simulink model "sym_uklad_D"  (R2024b)
settings: Solver=VariableStepAuto  StartTime=0.0  StopTime=0.01  RelTol=1e-3
settings Model: Creator=User  LastModifiedBy=User

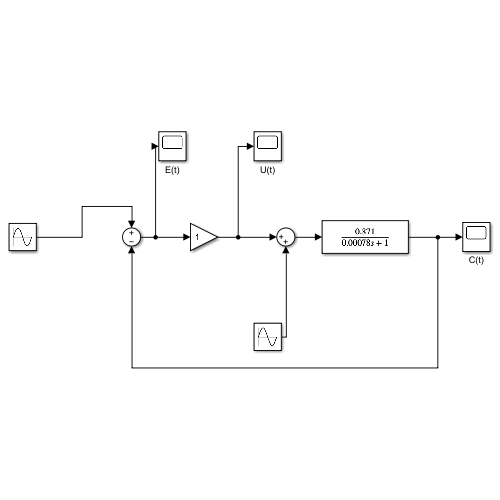
[thumbnail: Simulink's stored preview of the top-level diagram]
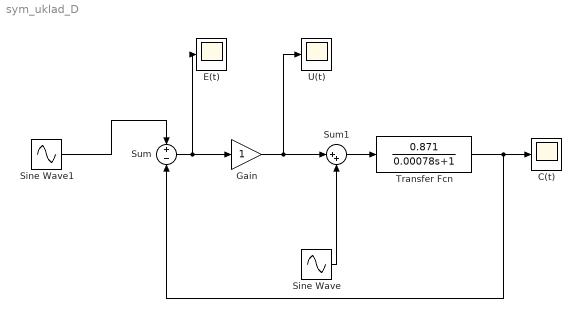
== system sym_uklad_D ==
  C(t) : Scope
  E(t) : Scope
  Gain : Gain
  Sine Wave : Sin  Frequency=300000  SampleTime=0
  Sine Wave1 : Sin  Amplitude=0  Frequency=10000  SampleTime=0
  Sum : Sum  Inputs=+-
  Sum1 : Sum  Inputs=|++
  Transfer Fcn : TransferFcn  Numerator=[0.871]  Denominator=[0.00078 1]
  U(t) : Scope
  wires:
  Gain/1 -> U(t)/1, Sum1/1
  Sum/1 -> E(t)/1, Gain/1
  Sum1/1 -> Transfer Fcn/1
  Transfer Fcn/1 -> Sum/2, C(t)/1
  Sine Wave1/1 -> Sum/1
  Sine Wave/1 -> Sum1/2
